simulink model "stm32f4_read_agm_imu_9a_host_demo"  (Simulink 7.3)
settings: Solver=ode45  StartTime=0.0  StopTime=inf  RelTol=1e-3
libraries: amg_usbconverter_n_connect_lib x2
settings Model: Creator=Krisada  LastModifiedBy=Krisada
settings HardwareCC: ProdEndianess=LittleEndian  ProdHWDeviceType=ARM Compatible->Cortex - M3  TargetEndianess=LittleEndian  TargetHWDeviceType=ARM Compatible->Cortex - M3
settings RTWCC: GenerateMakefile=off  ProcessScript=grt_make_rtw_hook

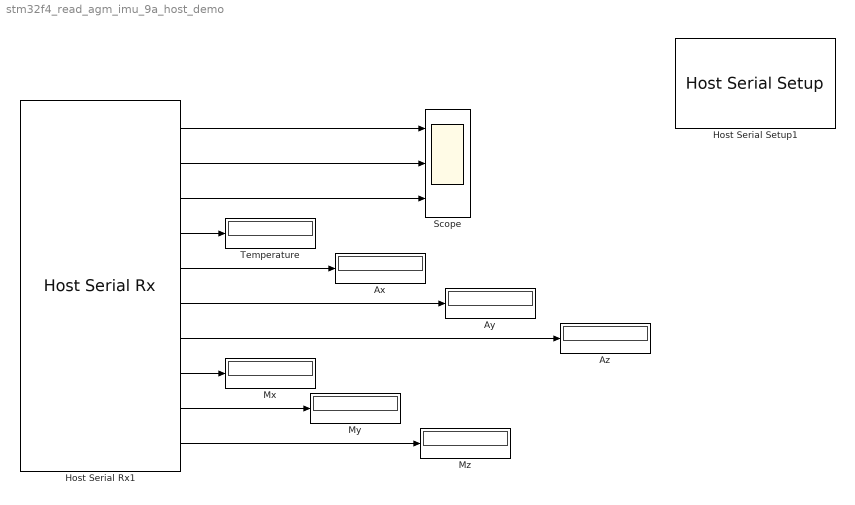
== system stm32f4_read_agm_imu_9a_host_demo ==
  Ax : Display
  Ay : Display
  Az : Display
  Host Serial Rx1 : amg_usbconverter_n_connect_lib/Host Serial Rx  conf=rx  port=<auto>  baudrate=115200  databits=8  parity=None  stopbit=1  flowcontrol=None  transfer=Blocking  timeout=5  packetmode=Binary  enableinitialvalues=off  initialvalues=[]  binheader='7E 7E'  binterminator='03 03'  porttype_double=0  porttype_single=10  porttype_int8=0  porttype_uint8=0  porttype_int16=0  porttype_uint16=0  porttype_int32=0  porttype_uint32=0  asciiformat='%d,%f'  rx_asciiterminator="CRLF (0x0D 0x0A - \"\\r\\n\")"  tx_asciiterminator="CRLF (0x0D 0x0A - \"\\r\\n\")"  sampletime=-1  enablecustomportlabel=off  cinputportlabel=0  coutputportlabel=A  portpinstr=0  blockid=HostSerialRx1  inputporttype=[]  inputportwidth=[]  inputportlabel={}  outputporttype=[1 1 1 1 1 1 1 1 1 1]  outputportwidth=[1 1 1 1 1 1 1 1 1 1]  outputportlabel={'single','single','single','single','single','single','single','single','single','single'}  compat=0  optionstring=[]  autoport='<empty>'
  Host Serial Setup1 : amg_usbconverter_n_connect_lib/Host Serial Setup  conf=setup  port=<auto>  baudrate=115200  databits=8  parity=None  stopbit=1  flowcontrol=None  transfer=Blocking  timeout=2  packetmode=Binary  initialvalues=[]  binheader='7E 7E'  binterminator='03 03'  porttype_double=0  porttype_single=1  porttype_int8=0  porttype_uint8=0  porttype_int16=0  porttype_uint16=0  porttype_int32=0  porttype_uint32=2  asciiformat='%d %u %x'  rx_asciiterminator="CRLF (0x0D 0x0A - \"\\r\\n\")"  tx_asciiterminator="CRLF (0x0D 0x0A - \"\\r\\n\")"  sampletime=-1  enablecustomportlabel=off  cinputportlabel=0  coutputportlabel=A  portpinstr=0  blockid=HostSerialSetup1  inputporttype=[]  inputportwidth=[]  inputportlabel={}  outputporttype=[]  outputportwidth=[]  outputportlabel={}  compat=0  optionstring=[]  autoport='<empty>'
  Mx : Display
  My : Display
  Mz : Display
  Scope : Scope  NumInputPorts=3
      settings: TimeRange=1200  YMin=-300~-300~-200  YMax=300~300~200
  Temperature : Display
  wires:
  Host Serial Rx1/1 -> Scope/1
  Host Serial Rx1/2 -> Scope/2
  Host Serial Rx1/3 -> Scope/3
  Host Serial Rx1/4 -> Temperature/1
  Host Serial Rx1/5 -> Ax/1
  Host Serial Rx1/6 -> Ay/1
  Host Serial Rx1/7 -> Az/1
  Host Serial Rx1/8 -> Mx/1
  Host Serial Rx1/9 -> My/1
  Host Serial Rx1/10 -> Mz/1
